simulink model "phdMain2"  (R2023b)
settings: Solver=ode4  StartTime=0.0  StopTime=t.Data(end)  FixedStep=1e-3  RelTol=1e-3
undefined symbols (not defined in the file): AEFF, Am, B_E, Bm, C_T, Cm, k, K, Kr0, Kx0, M, m3PsToLpm, PA_Pa, PaToBar, PB_Pa, PB_vec, V01, V02, V_DEAD, v_mPs, xc_dot, xc_m
(part 1 of 2)
settings Model: PauseTimes=22  Creator=snr  LastModifiedBy=snr
settings DataIOCC: OutputOption=AdditionalOutputTimes  OutputTimes=1
settings OptimizationCC: BlockReduction=off  ConditionallyExecuteInputs=off
settings DebuggingCC: UnderSpecifiedDimensionMsg=warning

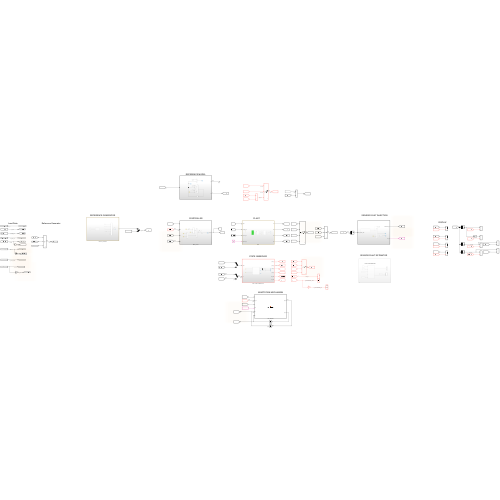
[thumbnail: Simulink's stored preview of the top-level diagram]
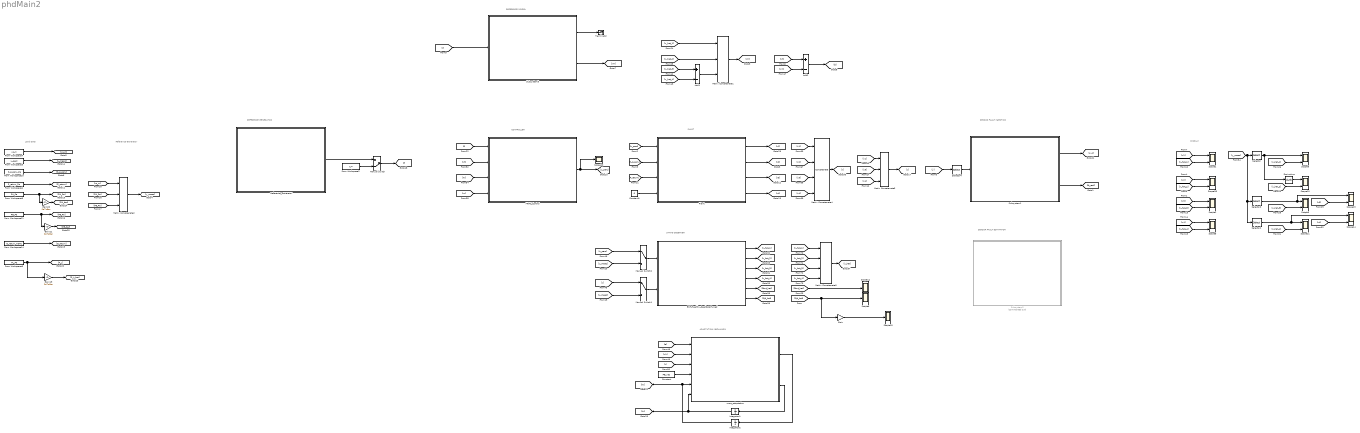
== system phdMain2 ==
  note: Load Data
  note: PLANT
  note: DISPLAY
  note: Reference Generator
  note: SENSOR FAULT INJECTION
  note: STATE OBSERVER
  note: SENSOR FAULT ESTIMATOR
  note: REFERENCE GENERATOR
  note: REFERENCE MODEL
  note: ADAPTATION MECHANISM
  note: CONTROLLER
  Add1 : Sum  Inputs=+-
  Add2 : Sum  Inputs=+-
  Constant : Constant  Value=PB_vec
  Constant1 : Constant  Value=0
  Derivative : Derivative
  EKF_Healthy_RealDataTuned : Subsystem
  From Workspace1 : FromWorkspace  VariableName=P_return_Pa
  From Workspace10 : FromWorkspace  VariableName=P_supply_Pa
  From Workspace11 : FromWorkspace  VariableName=PB_Pa
  From Workspace14 : FromWorkspace  VariableName=Q_return_m3Ps
  From Workspace2 : FromWorkspace  VariableName=r_m
  From Workspace3 : FromWorkspace  VariableName=u_perc
  From Workspace4 : FromWorkspace  VariableName=xc_m
  From Workspace5 : FromWorkspace  VariableName=PL_Pa
  From Workspace9 : FromWorkspace  VariableName=PA_Pa
  Gain : Gain  Gain=60e3
  Gain19 : Gain  Gain=PaToBar
  Gain20 : Gain  Gain=PaToBar
  Gain21 : Gain  Gain=PaToBar
  Integrator1 : Integrator  InitialCondition=Kr0
  Integrator2 : Integrator  InitialCondition=Kx0
  MRAC_Control : Subsystem
  Manual Switch : ManualSwitch  CurrentSetting=0
  Manual Switch1 : ManualSwitch
  Manual Switch2 : ManualSwitch
  Matrix Concatenate1 : Concatenate  NumInputs=3  Mode=Multidimensional array
  Matrix Concatenate2 : Concatenate  NumInputs=3  Mode=Multidimensional array
  Matrix Concatenate3 : Concatenate  NumInputs=3  Mode=Multidimensional array
  Matrix Concatenate4 : Concatenate  NumInputs=4  Mode=Multidimensional array
  Matrix Concatenate5 : Concatenate  NumInputs=4  Mode=Multidimensional array
  Plant : Subsystem
  Reference_Generator : Subsystem
  Scope{1..2,5,8..11,13..14,36} (10 alike) : Scope  NumInputPorts=2
  Scope{6,12,15,20} (4 alike) : Scope
  Selector : Selector  InputPortWidth=3  IndexOptions=Index vector (dialog)  Indices=1  OutputSizes=1
  Selector1 : Selector  InputPortWidth=3  IndexOptions=Index vector (dialog)  Indices=3  OutputSizes=1
  Selector2 : Selector  InputPortWidth=3  IndexOptions=Index vector (dialog)  Indices=2  OutputSizes=1
  Selector4 : Selector  InputPortWidth=3  IndexOptions=Index vector (dialog)  Indices=1  OutputSizes=1
  Subsystem1 : Subsystem
  Subsystem2 : Subsystem  Commented=on
  Subsystem3 : Subsystem
  Terminator : Terminator
  mrac_adaptation : MATLAB Function  TreatAsAtomicUnit=on
  wires:
  From Workspace3/1 -> [u_meas]  "u_real"
  From Workspace10/1 -> [P_supply]  "P_supply_Pa"
  From Workspace1/1 -> [P_return]  "P_return_Pa"
  From Workspace9/1 -> Gain20/1, [PA_Pa]  "PA_Pa"
  From Workspace11/1 -> Gain21/1, [PB_Pa]  "PB_Pa"
  From Workspace14/1 -> [Q_return]  "Q_return_m3Ps"
  From Workspace5/1 -> [P_L], Gain19/1  "P_L_Pa"
  Gain19/1 -> [P_L_bar]  "P_L_bar"
  Gain20/1 -> [PA_bar]  "PA_bar"
  Gain21/1 -> [PB_bar]  "PB_bar"
  [P_supply] -> Plant/2(P_supply_Pa)
  [P_return] -> Plant/3(P_return_Pa)
  Plant/1(x1) -> [x1]
  Plant/2(x2) -> [x2]
  Plant/3(x3) -> [x3]
  Plant/4(x4) -> [x4]
  [x1] -> Matrix Concatenate3/1
  [x3] -> Matrix Concatenate3/2
  [x4] -> Matrix Concatenate3/3
  Matrix Concatenate3/1 -> [y]
  EKF_Healthy_RealDataTuned/1(x_hat_1) -> [x_hat_1]  "x_hat_1"
  EKF_Healthy_RealDataTuned/2(x_hat_2) -> [x_hat_2]  "x_hat_2"
  EKF_Healthy_RealDataTuned/3(x_hat_3) -> [x_hat_3]
  EKF_Healthy_RealDataTuned/4(x_hat_4) -> [x_hat_4]
  [x1] -> Matrix Concatenate4/1
  [x2] -> Matrix Concatenate4/2
  [x3] -> Matrix Concatenate4/3
  [x4] -> Matrix Concatenate4/4
  Matrix Concatenate4/1 -> [x]
  [x_hat_1] -> Matrix Concatenate5/1
  [x_hat_2] -> Matrix Concatenate5/2
  [x_hat_3] -> Matrix Concatenate5/3
  [x_hat_4] -> Matrix Concatenate5/4
  Matrix Concatenate5/1 -> [x_hat]
  EKF_Healthy_RealDataTuned/5(Fext_hat) -> [Fext_hat]
  EKF_Healthy_RealDataTuned/6(Qd_est) -> [Qd_hat]
  [x2] -> Scope36/1
  [x_hat_2] -> Scope36/2
  [y] -> Selector4/1
  Selector4/1 -> Subsystem1/1(Real_Cylinder_Pos)
  Subsystem1/1(Measured_Pos) -> [y_1]
  Subsystem1/2(fs_real) -> [fs_real]
  [r] -> Subsystem3/1(r)  "r"
  Manual Switch/1 -> [r]  "r_m"
  Reference_Generator/1(r) -> Manual Switch/1  "r"
  From Workspace2/1 -> Manual Switch/2
  [x1] -> Scope1/1
  [x_hat_1] -> Scope1/2
  [x_hat_3] -> Scope2/2
  [x3] -> Scope2/1
  [x4] -> Scope5/1
  [x_hat_4] -> Scope5/2
  [Qd_hat] -> Gain/1, Scope6/1  "Q_unmodeledLeak_m3Ps"
  [PB_Pa] -> Matrix Concatenate2/3
  [PA_Pa] -> Matrix Concatenate2/2
  [xc_m] -> Matrix Concatenate2/1
  Matrix Concatenate2/1 -> [y_meas]
  Manual Switch1/1 -> EKF_Healthy_RealDataTuned/2(y_k)
  [y] -> Manual Switch1/1
  [y_meas] -> Manual Switch1/2
  Manual Switch2/1 -> EKF_Healthy_RealDataTuned/1(u_perc)
  [u_perc] -> Manual Switch2/1
  [u_meas] -> Manual Switch2/2
  [u_perc] -> Plant/1(u_perc)
  Selector1/1 -> Scope14/1, Scope11/1  "P2_real"
  [x_hat_4] -> Scope11/2
  Selector/1 -> Derivative/1, Scope8/1
  [x_hat_1] -> Scope8/2
  [x_hat_2] -> Scope10/2
  Derivative/1 -> Scope10/1
  [x_hat_3] -> Scope9/2
  Selector2/1 -> Scope13/1, Scope9/1  "P1_real"
  [y_meas] -> Selector1/1, Selector2/1, Selector/1
  From Workspace4/1 -> [xc_m]  "xc_m"
  [Fext_hat] -> Scope12/1  "Fext_N"
  [x3] -> Scope13/2
  [x4] -> Scope14/2
  Gain/1 -> Scope15/1  "Q_unmodeledLeak_lpm"
  Subsystem3/1(ym) -> Terminator/1
  Subsystem3/2(xm) -> [xm]
  [x_hat_3] -> Add1/1
  [x_hat_4] -> Add1/2
  Add1/1 -> Matrix Concatenate1/3  "PL_hat"
  [x_hat_2] -> Matrix Concatenate1/2  "x2_hat"
  [x_hat_1] -> Matrix Concatenate1/1  "x1_hat"
  Add2/1 -> [e]  "e"
  [xm] -> Add2/2
  Matrix Concatenate1/1 -> [xh]
  [e] -> mrac_adaptation/1(e)
  [xh] -> mrac_adaptation/2(x_hat)
  [r] -> mrac_adaptation/3(r)
  mrac_adaptation/2(Kr_dot) -> Integrator1/1
  Integrator1/1 -> [Kr], mrac_adaptation/6(Kr)
  mrac_adaptation/1(Kx_dot) -> Integrator2/1
  Integrator2/1 -> mrac_adaptation/5(Kx), [Kx]
  Constant/1 -> mrac_adaptation/4(PB)
  [r] -> MRAC_Control/1(r)
  [xx] -> MRAC_Control/4(xh)
  MRAC_Control/1(u_out_perc) -> Scope20/1, [u_perc]
  [xh] -> MRAC_Control/2(Kx)
  [Kr] -> MRAC_Control/3(Kr)
  Constant1/1 -> Plant/4(F_external_N)
  [xh] -> Add2/1

== system phdMain2/EKF_Healthy_RealDataTuned ==
  u_perc : Inport  OutDataTypeStr=double
  y_k : Inport  Port=2  OutDataTypeStr=double
  EKF_Discrete : MATLAB Function  TreatAsAtomicUnit=on  SystemSampleTime=1e-3
  Sel_d10 : Selector  InputPortWidth=6  IndexOptions=Index vector (dialog)  Indices=4  OutputSizes=1
  Sel_d7 : Selector  InputPortWidth=6  IndexOptions=Index vector (dialog)  Indices=1  OutputSizes=1
  Sel_d8 : Selector  InputPortWidth=6  IndexOptions=Index vector (dialog)  Indices=2  OutputSizes=1  RuntimeRangeChecks=on
  Sel_d9 : Selector  InputPortWidth=6  IndexOptions=Index vector (dialog)  Indices=3  OutputSizes=1
  Unit Delay : UnitDelay  SampleTime=1e-3  HasFrameUpgradeWarning=on
  x_hat_1 : Outport  OutDataTypeStr=double
  x_hat_2 : Outport  Port=2  OutDataTypeStr=double
  x_hat_3 : Outport  Port=3  OutDataTypeStr=double
  x_hat_4 : Outport  Port=4  OutDataTypeStr=double
  Fext_hat : Outport  Port=5  OutDataTypeStr=double
  Qd_est : Outport  Port=6  OutDataTypeStr=double
  wires:
  u_perc/1 -> EKF_Discrete/1(u_perc)  "u_perc"
  y_k/1 -> EKF_Discrete/2(y_k)
  EKF_Discrete/1(x_hat_out) -> Unit Delay/1
  Sel_d7/1 -> x_hat_1/1  "x_hat_1"
  Sel_d8/1 -> x_hat_2/1  "x_hat_2"
  Sel_d9/1 -> x_hat_3/1  "x_hat_3"
  Sel_d10/1 -> x_hat_4/1  "x_hat_4"
  EKF_Discrete/2(Fd_est) -> Fext_hat/1
  EKF_Discrete/3(Qd_est) -> Qd_est/1
  Unit Delay/1 -> Sel_d7/1, Sel_d10/1, Sel_d9/1, Sel_d8/1

== system phdMain2/MRAC_Control ==
  r : Inport  OutDataTypeStr=double
  Kx : Inport  Port=2  OutDataTypeStr=double
  Kr : Inport  Port=3  OutDataTypeStr=double
  xh : Inport  Port=4  OutDataTypeStr=double
  Add : Sum
  Product : Product  Multiplication=Matrix(*)
  Product1 : Product  Multiplication=Matrix(*)
  Saturation : Saturate  UpperLimit=100  LowerLimit=-100
  Scope : Scope
  Transpose : Math  Operator=transpose
  u_out_perc : Outport  OutDataTypeStr=double
  wires:
  xh/1 -> Product/2
  Kx/1 -> Transpose/1
  Transpose/1 -> Product/1
  r/1 -> Product1/2
  Kr/1 -> Product1/1
  Product1/1 -> Add/2
  Product/1 -> Add/1
  Add/1 -> Scope/1, Saturation/1
  Saturation/1 -> u_out_perc/1

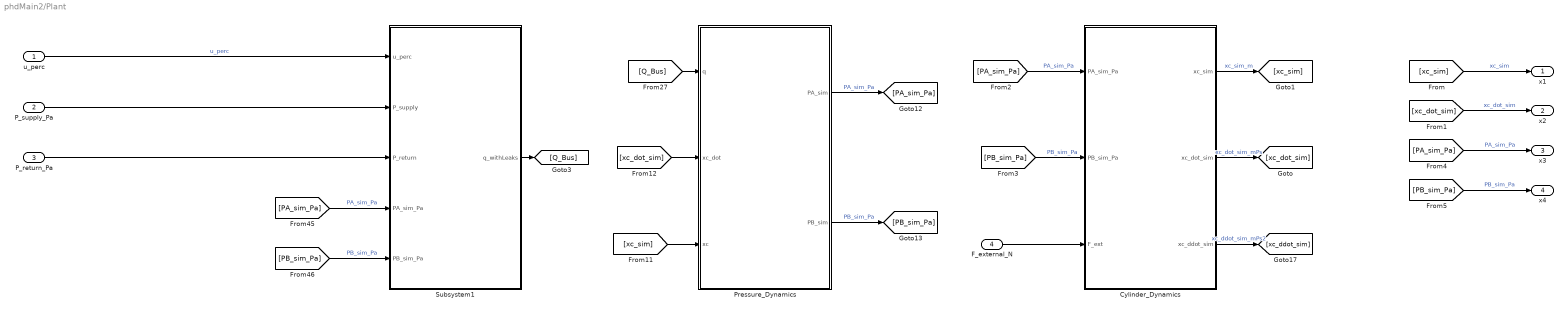
== system phdMain2/Plant ==
  u_perc : Inport  OutDataTypeStr=double
  P_supply_Pa : Inport  Port=2
  P_return_Pa : Inport  Port=3
  F_external_N : Inport  Port=4
  Cylinder_Dynamics : Subsystem
  Pressure_Dynamics : Subsystem
  Subsystem1 : Subsystem
  x1 : Outport
  x2 : Outport  Port=2
  x3 : Outport  Port=3
  x4 : Outport  Port=4
  wires:
  Cylinder_Dynamics/1(xc_sim) -> [xc_sim]  "xc_sim_m"
  [xc_sim] -> Pressure_Dynamics/3(xc)
  P_supply_Pa/1 -> Subsystem1/2(P_supply)
  [PA_sim_Pa] -> Subsystem1/4(PA_sim_Pa)  "PA_sim_Pa"
  [PB_sim_Pa] -> Subsystem1/5(PB_sim_Pa)  "PB_sim_Pa"
  [PB_sim_Pa] -> Cylinder_Dynamics/2(PB_sim_Pa)  "PB_sim_Pa"
  Pressure_Dynamics/1(PA_sim) -> [PA_sim_Pa]  "PA_sim_Pa"
  Cylinder_Dynamics/3(xc_ddot_sim) -> [xc_ddot_sim]  "xc_ddot_sim_mPs2"
  Cylinder_Dynamics/2(xc_dot_sim) -> [xc_dot_sim]  "xc_dot_sim_mPs"
  [xc_dot_sim] -> Pressure_Dynamics/2(xc_dot)
  [PA_sim_Pa] -> Cylinder_Dynamics/1(PA_sim_Pa)  "PA_sim_Pa"
  Pressure_Dynamics/2(PB_sim) -> [PB_sim_Pa]  "PB_sim_Pa"
  Subsystem1/1(q_withLeaks) -> [Q_Bus]
  [Q_Bus] -> Pressure_Dynamics/1(q)
  u_perc/1 -> Subsystem1/1(u_perc)  "u_perc"
  P_return_Pa/1 -> Subsystem1/3(P_return)
  F_external_N/1 -> Cylinder_Dynamics/3(F_ext)
  [xc_sim] -> x1/1  "xc_sim"
  [xc_dot_sim] -> x2/1  "xc_dot_sim"
  [PA_sim_Pa] -> x3/1  "PA_sim_Pa"
  [PB_sim_Pa] -> x4/1  "PB_sim_Pa"

== system phdMain2/Reference_Generator ==
  Constant : Constant  OutDataTypeStr=uint8
  Constant1 : Constant  Commented=on  Value=30  OutDataTypeStr=double
  Constant2 : Constant  Commented=on  OutDataTypeStr=double
  Constant3 : Constant  Commented=on  Value=0  OutDataTypeStr=double
  Constant4 : Constant  Value=0
  From Workspace14 : FromWorkspace  VariableName=r_m
  Gain : Gain
  Multiport Switch : MultiPortSwitch  DataPortOrder=Zero-based contiguous  DataPortForDefault=Additional data port  DiagnosticForDefault=None  zeroidx=on  OutDataTypeStr=double  SaturateOnIntegerOverflow=off  InputSameDT=off
  Pulse Generator : DiscretePulseGenerator  PulseType=Time based  Amplitude=20e-3  Period=4  PulseWidth=25
  Scope : Scope
  Sine Wave : Sin  Amplitude=30e-3  Frequency=pi*0.5  SampleTime=0
  Sine_Generator : Subsystem  Commented=on
  r : Outport  OutDataTypeStr=double
  wires:
  From Workspace14/1 -> Multiport Switch/2  "r_m"
  Constant/1 -> Multiport Switch/1
  Constant1/1 -> Sine_Generator/1(Amp_mm)
  Constant2/1 -> Sine_Generator/2(f_Hz)
  Constant3/1 -> Sine_Generator/3(phi_deg)
  Pulse Generator/1 -> Gain/1
  Multiport Switch/1 -> Scope/1, r/1
  Constant4/1 -> Multiport Switch/5
  Sine Wave/1 -> Multiport Switch/3
  Gain/1 -> Multiport Switch/4

== system phdMain2/Subsystem1 ==
  Real_Cylinder_Pos : Inport  OutDataTypeStr=double
  Add4 : Sum
  Fault_Injection : Subsystem  Commented=on
  Measured_Pos : Outport  OutDataTypeStr=double
  fs_real : Outport  Port=2  OutDataTypeStr=double
  wires:
  Fault_Injection/1(fs) -> [fs_real], Add4/1
  Real_Cylinder_Pos/1 -> Add4/2
  Add4/1 -> Measured_Pos/1  "y_1"
  [fs_real] -> fs_real/1

== system phdMain2/Subsystem2 ==
  note: FAULT ESTIMATOR
  From14 : From  Commented=on  GotoTag=u_perc
  From15 : From  Commented=on  GotoTag=PA_sim_Pa
  From20 : From  Commented=on  GotoTag=PB_sim_Pa
  From29 : From  Commented=on  GotoTag=fs_real
  From33 : From  Commented=on  GotoTag=xc_dot_sim
  Scope12 : Scope  Commented=on  NumInputPorts=3
  Scope17 : Scope  Commented=on  NumInputPorts=3
  Subsystem3 : Subsystem  Commented=on
  wires:
  Subsystem3/2(Out1) -> Scope17/1
  From20/1 -> Subsystem3/3(PB_Pa)  "PB_sim_Pa"
  From29/1 -> Subsystem3/5(fs_real)
  From14/1 -> Subsystem3/1(u_real)  "u_perc"
  From33/1 -> Scope17/2
  From15/1 -> Subsystem3/2(PA_Pa)
  Subsystem3/1(x_bar) -> Scope12/2  "x_bar"

== system phdMain2/Subsystem3 ==
  r : Inport  OutDataTypeStr=double
  Add : Sum
  Constant : Constant  Value=Am
  Constant1 : Constant  Value=Bm
  Constant2 : Constant  Value=Cm
  Integrator1 : Integrator  InitialCondition=[0;0;0]
  Product : Product  Multiplication=Matrix(*)
  Product1 : Product  Multiplication=Matrix(*)
  Product2 : Product  Multiplication=Matrix(*)
  ym : Outport  OutDataTypeStr=double  PortDimensions=[3,1]
  xm : Outport  Port=2  OutDataTypeStr=double
  wires:
  Constant/1 -> Product/1
  Constant1/1 -> Product1/1
  r/1 -> Product1/2  "r"
  Product1/1 -> Add/2
  Product/1 -> Add/1
  Add/1 -> Integrator1/1  "dxm"
  Integrator1/1 -> Product/2, Product2/2, xm/1  "xm"
  Product2/1 -> ym/1
  Constant2/1 -> Product2/1

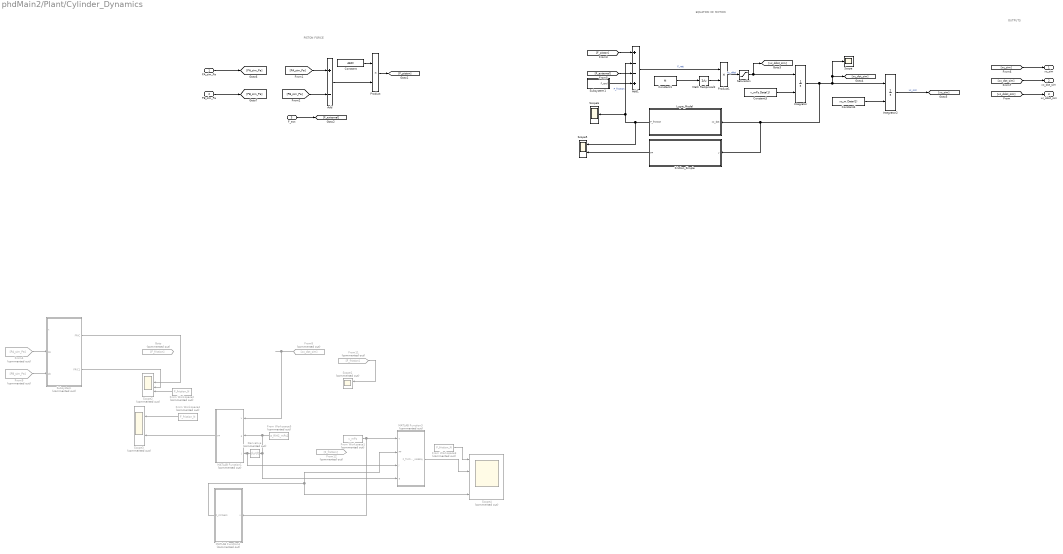
== system phdMain2/Plant/Cylinder_Dynamics ==
  note: PISTON FORCE
  note: EQUATION OF MOTION
  note: OUTPUTS
  PA_sim_Pa : Inport  OutDataTypeStr=double
  PB_sim_Pa : Inport  Port=2  OutDataTypeStr=double
  F_ext : Inport  Port=3  OutDataTypeStr=double
  Add : Sum  Inputs=+-
  Add1 : Sum  Inputs=+--+
  Constant : Constant  Value=AEFF  OutDataTypeStr=double
  Constant1 : Constant  Value=M  OutDataTypeStr=double
  Constant3 : Constant  Value=v_mPs.Data(1)
  Constant4 : Constant  Value=xc_m.Data(1)
  Derivative : Derivative  Commented=on
  Friction_Simple : MATLAB Function  TreatAsAtomicUnit=on
  From Workspace1 : FromWorkspace  Commented=on  VariableName=v_mPs
  From Workspace2 : FromWorkspace  Commented=on  VariableName=F_friction_N
  From Workspace3 : FromWorkspace  Commented=on  VariableName=F_friction_N
  From Workspace4 : FromWorkspace  Commented=on  VariableName=F_friction_N
  From Workspace5 : FromWorkspace  Commented=on  VariableName=a_RMC_mPs2
  From11 : From  Commented=on  GotoTag=F_friction
  From12 : From  Commented=on  GotoTag=F_friction
  From4 : From  Commented=on  GotoTag=PA_sim_Pa
  From8 : From  Commented=on  GotoTag=xc_dot_sim
  From9 : From  Commented=on  GotoTag=PB_sim_Pa
  Goto : Goto  Commented=on  GotoTag=F_friction
  Integrator : Integrator  InitialConditionSource=external  InitialCondition=xc_dot(1)  UpperSaturationLimit=4  LowerSaturationLimit=-4
  Integrator2 : Integrator  InitialConditionSource=external  InitialCondition=xc_dot(1)  LimitOutput=on  UpperSaturationLimit=0.09580  LowerSaturationLimit=-0.09580
  Lugre_Model : Subsystem
  MATLAB Function1 : MATLAB Function  Commented=on  TreatAsAtomicUnit=on
  MATLAB Function3 : MATLAB Function  Commented=on  TreatAsAtomicUnit=on
  MATLAB Function4 : MATLAB Function  Commented=on  TreatAsAtomicUnit=on
  Math Reciprocal2 : Math  Operator=reciprocal  SignedPower=on
  Product : Product
  Product1 : Product
  Saturation : Saturate  UpperLimit=100  LowerLimit=-100
  Scope : Scope
  Scope1 : Scope  Commented=on  NumInputPorts=2
  Scope2 : Scope  Commented=on  NumInputPorts=6
  Scope3 : Scope  Commented=on  NumInputPorts=2
  Scope4 : Scope  Commented=on  NumInputPorts=4
  Scope5 : Scope  NumInputPorts=2
  Scope6 : Scope
  Subsystem : Subsystem  Commented=on
  Subsystem1 : Subsystem
  xc_sim : Outport  OutDataTypeStr=double
  xc_dot_sim : Outport  Port=2  OutDataTypeStr=double
  xc_ddot_sim : Outport  Port=3  OutDataTypeStr=double
  wires:
  [PB_sim_Pa] -> Add/2
  [PA_sim_Pa] -> Add/1
  Add/1 -> Product/2
  Constant/1 -> Product/1
  Math Reciprocal2/1 -> Product1/2
  Product1/1 -> Saturation/1  "xc_ddot"
  Product/1 -> [F_piston]
  F_ext/1 -> [F_external]
  Add1/1 -> Product1/1  "F_net"
  Constant3/1 -> Integrator/2
  Integrator/1 -> Integrator2/1, Scope/1, [xc_dot_sim], Friction_Simple/1(v), Lugre_Model/1(xc_dot)
  Constant4/1 -> Integrator2/2
  Integrator2/1 -> [xc_sim]  "xc_sim"
  [xc_sim] -> xc_sim/1
  [xc_dot_sim] -> xc_dot_sim/1
  From8/1 -> MATLAB Function1/1(v)
  [xc_ddot_sim] -> xc_ddot_sim/1
  Saturation/1 -> [xc_ddot_sim], Integrator/1
  [F_external] -> Add1/3
  [F_piston] -> Add1/1
  ? -> Scope2/1, Goto/1  "F_friction"
  From Workspace2/1 -> Scope2/5
  Subsystem1/1(F_end) -> Add1/4
  PA_sim_Pa/1 -> [PA_sim_Pa]
  PB_sim_Pa/1 -> [PB_sim_Pa]
  From4/1 -> Subsystem/2(pa)
  From9/1 -> Subsystem/3(pb)
  Constant1/1 -> Math Reciprocal2/1
  Subsystem/2(FRIC1) -> Scope2/4
  Subsystem/1(FRIC) -> Scope2/3
  Derivative/1 -> MATLAB Function3/3(j), MATLAB Function1/3(j)
  From Workspace4/1 -> Scope3/1
  MATLAB Function1/1(FF) -> Scope3/2
  From Workspace5/1 -> MATLAB Function3/4(a), Derivative/1, MATLAB Function1/2(a)
  From11/1 -> Scope1/1
  From Workspace1/1 -> MATLAB Function4/1(v), MATLAB Function3/1(v)
  MATLAB Function3/1(F_friction_nodelay) -> Scope4/2
  From Workspace3/1 -> Scope4/1
  MATLAB Function4/1(F_stribeck) -> MATLAB Function3/2(FF), Scope4/4
  Lugre_Model/1(F_friction) -> Add1/2, Scope6/1, Scope5/1  "F_friction"
  Friction_Simple/1(FF) -> Scope5/2

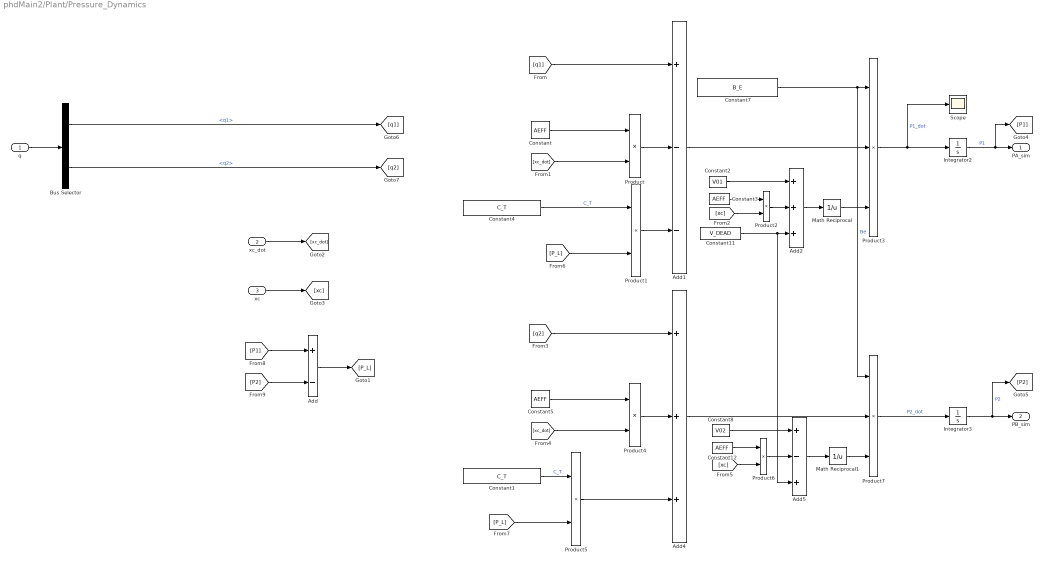
== system phdMain2/Plant/Pressure_Dynamics ==
  q : Inport  OutDataTypeStr=double
  xc_dot : Inport  Port=2  OutDataTypeStr=double
  xc : Inport  Port=3  OutDataTypeStr=double
  Add : Sum  Inputs=+-
  Add1 : Sum  Inputs=+--
  Add2 : Sum  Inputs=+++
  Add4 : Sum  Inputs=+++
  Add5 : Sum  Inputs=+-+
  Bus Selector : BusSelector  OutputSignals=q1,q2
  Constant{,3,5,12} (4 alike) : Constant  Value=AEFF  OutDataTypeStr=double
  Constant1 : Constant  Value=C_T  OutDataTypeStr=double
  Constant11 : Constant  Value=V_DEAD  OutDataTypeStr=double
  Constant2 : Constant  Value=V01  OutDataTypeStr=double
  Constant4 : Constant  Value=C_T  OutDataTypeStr=double
  Constant7 : Constant  Value=B_E  OutDataTypeStr=double
  Constant8 : Constant  Value=V02  OutDataTypeStr=double
  Integrator2 : Integrator  InitialCondition=PA_Pa.Data(1)  LimitOutput=on  UpperSaturationLimit=200e5  LowerSaturationLimit=4e5
  Integrator3 : Integrator  InitialCondition=PB_Pa.Data(1)  LimitOutput=on  UpperSaturationLimit=200e5  LowerSaturationLimit=4e5
  Math Reciprocal : Math  Operator=reciprocal  SignedPower=on
  Math Reciprocal1 : Math  Operator=reciprocal  SignedPower=on
  Product{,1..2,4..6} (6 alike) : Product
  Product3 : Product  Inputs=3
  Product7 : Product  Inputs=3
  Scope : Scope
  PA_sim : Outport  OutDataTypeStr=double
  PB_sim : Outport  Port=2  OutDataTypeStr=double
  wires:
  q/1 -> Bus Selector/1
  xc_dot/1 -> [xc_dot]
  [xc_dot] -> Product/2
  Constant/1 -> Product/1
  Integrator2/1 -> [P1], PA_sim/1  "P1"
  [P_L] -> Product1/2
  Product/1 -> Add1/2
  [q1] -> Add1/1
  xc/1 -> [xc]
  Constant2/1 -> Add2/1
  Product2/1 -> Add2/2
  [xc] -> Product2/2
  Constant3/1 -> Product2/1
  Add2/1 -> Math Reciprocal/1
  Product3/1 -> Integrator2/1, Scope/1  "P1_dot"
  Math Reciprocal/1 -> Product3/3
  Add1/1 -> Product3/2
  Constant7/1 -> Product7/1, Product3/1  "Be"
  Constant4/1 -> Product1/1  "C_T"
  [xc_dot] -> Product4/2
  Product4/1 -> Add4/2
  Add4/1 -> Product7/2
  Integrator3/1 -> [P2], PB_sim/1  "P2"
  [P_L] -> Product5/2
  Constant5/1 -> Product4/1
  Add5/1 -> Math Reciprocal1/1
  [q2] -> Add4/1
  Math Reciprocal1/1 -> Product7/3
  Product7/1 -> Integrator3/1  "P2_dot"
  [xc] -> Product6/2
  Constant8/1 -> Add5/1
  Constant12/1 -> Product6/1
  Product6/1 -> Add5/2
  Bus Selector/2 -> [q2]  "<q2>"
  Bus Selector/1 -> [q1]  "<q1>"
  [P2] -> Add/2
  [P1] -> Add/1
  Add/1 -> [P_L]
  Constant1/1 -> Product5/1  "C_T"
  Product5/1 -> Add4/3
  Product1/1 -> Add1/3
  Constant11/1 -> Add5/3, Add2/3

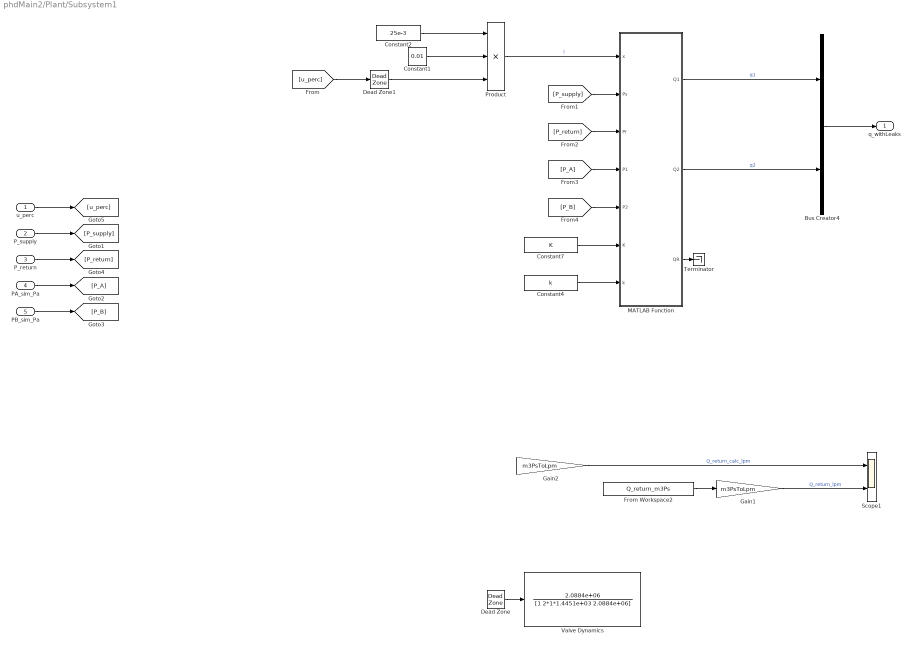
== system phdMain2/Plant/Subsystem1 ==
  u_perc : Inport  OutDataTypeStr=double
  P_supply : Inport  Port=2  OutDataTypeStr=double
  P_return : Inport  Port=3  OutDataTypeStr=double
  PA_sim_Pa : Inport  Port=4  OutDataTypeStr=double
  PB_sim_Pa : Inport  Port=5  OutDataTypeStr=double
  Bus Creator4 : BusCreator  Inputs=2
  Constant1 : Constant  Value=0.01
  Constant2 : Constant  Value=25e-3
  Constant4 : Constant  Value=k
  Constant7 : Constant  Value=K
  Dead Zone : DeadZone  LowerValue=-0.02  UpperValue=0.02
  Dead Zone1 : DeadZone  LowerValue=-0.02  UpperValue=0.02
  From Workspace2 : FromWorkspace  VariableName=Q_return_m3Ps
  Gain1 : Gain  Gain=m3PsToLpm
  Gain2 : Gain  Gain=m3PsToLpm
  MATLAB Function : MATLAB Function  TreatAsAtomicUnit=on
  Product : Product  Inputs=3
  Scope1 : Scope  NumInputPorts=2
  Terminator : Terminator
  Valve Dynamics : TransferFcn  Numerator=[2.0884e+06]  Denominator=[1 2*1*1.4451e+03 2.0884e+06]
  q_withLeaks : Outport  OutDataTypeStr=double
  wires:
  PA_sim_Pa/1 -> [P_A]
  P_supply/1 -> [P_supply]
  P_return/1 -> [P_return]
  PB_sim_Pa/1 -> [P_B]
  u_perc/1 -> [u_perc]
  [P_supply] -> MATLAB Function/2(Ps)
  [P_return] -> MATLAB Function/3(Pr)
  [P_A] -> MATLAB Function/4(P1)
  [P_B] -> MATLAB Function/5(P2)
  Bus Creator4/1 -> q_withLeaks/1
  MATLAB Function/1(Q1) -> Bus Creator4/1  "q1"
  MATLAB Function/2(Q2) -> Bus Creator4/2  "q2"
  Constant2/1 -> Product/1
  Product/1 -> MATLAB Function/1(x)  "i"
  Constant1/1 -> Product/2
  Constant4/1 -> MATLAB Function/7(k)
  Constant7/1 -> MATLAB Function/6(K)
  [u_perc] -> Dead Zone1/1
  From Workspace2/1 -> Gain1/1
  Gain2/1 -> Scope1/1  "Q_return_calc_lpm"
  Gain1/1 -> Scope1/2  "Q_return_lpm"
  MATLAB Function/3(QR) -> Terminator/1
  Dead Zone/1 -> Valve Dynamics/1
  Dead Zone1/1 -> Product/3

== system phdMain2/Reference_Generator/Sine_Generator ==
  Amp_mm : Inport  OutDataTypeStr=double
  f_Hz : Inport  Port=2
  phi_deg : Inport  Port=3  OutDataTypeStr=double
  Add : Sum
  Clock : Clock
  Constant : Constant  Value=2
  Constant1 : Constant  Value=3.14159265359
  Constant2 : Constant  Value=3.14159265359
  Constant3 : Constant  Value=180
  Constant4 : Constant  Value=1e-3
  Math Reciprocal : Math  Operator=reciprocal  SignedPower=on
  Product : Product  Inputs=4
  Product{1..4} (4 alike) : Product
  Sin : Trigonometry
  r : Outport
  wires:
  Constant1/1 -> Product/2
  Constant/1 -> Product/1
  f_Hz/1 -> Product/3
  phi_deg/1 -> Product1/1
  Constant2/1 -> Product2/1
  Constant3/1 -> Math Reciprocal/1
  Math Reciprocal/1 -> Product2/2
  Product2/1 -> Product1/2
  Clock/1 -> Product/4
  Product/1 -> Sin/1
  Sin/1 -> Product3/2
  Product1/1 -> Add/2
  Product3/1 -> Add/1
  Add/1 -> r/1
  Amp_mm/1 -> Product4/2
  Product4/1 -> Product3/1
  Constant4/1 -> Product4/1

== system phdMain2/Subsystem1/Fault_Injection ==
  Constant : Constant  Value=0
  fs : Outport  OutDataTypeStr=double
  wires:
  Constant/1 -> fs/1

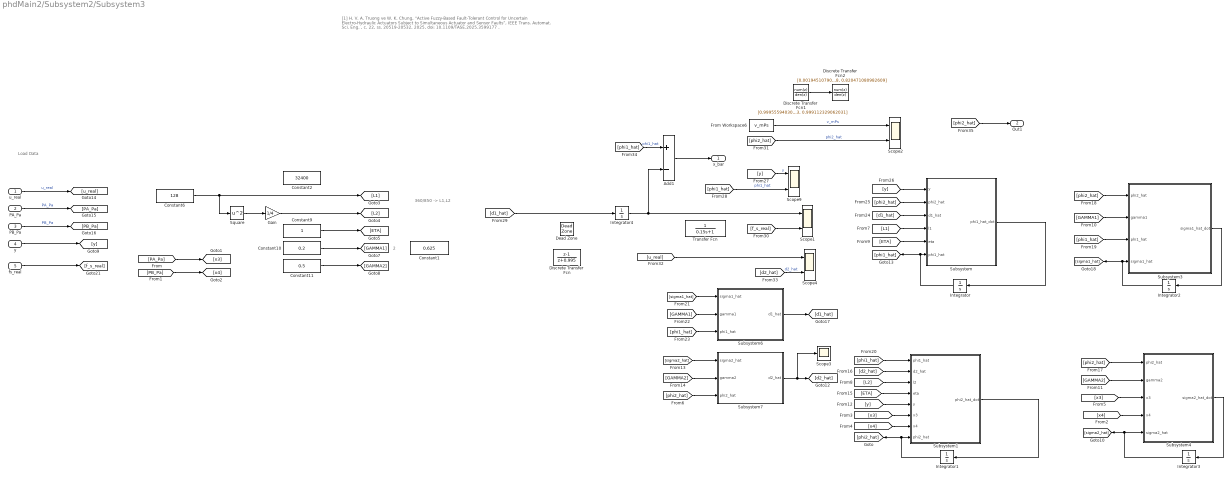
== system phdMain2/Subsystem2/Subsystem3 ==
  note: [1]
      | H. V. A. Truong ve W. K. Chung, “Active Fuzzy-Based Fault-Tolerant Control for Uncertain Electro-Hydraulic Actuators Subject to Simultaneous Actuator and Sensor Faults”, IEEE Trans. Automat. Sci. Eng. , c. 22, ss. 20519-20532, 2025, doi: 10.1109/TASE.2025.3599177 .
  note: 2
  note: 360/850 -> L1,L2
  note: Load Data
  u_real : Inport
  PA_Pa : Inport  Port=2
  PB_Pa : Inport  Port=3
  y : Inport  Port=4
  fs_real : Inport  Port=5
  Add1 : Sum  Inputs=+-
  Constant1 : Constant  Value=0.625
  Constant10 : Constant  Value=0.2
  Constant11 : Constant  Value=0.5
  Constant2 : Constant  Value=32400
  Constant6 : Constant  Value=128
  Constant9 : Constant
  Dead Zone : DeadZone  LowerValue=-0.01  UpperValue=0.01
  Discrete Transfer Fcn : DiscreteTransferFcn  Numerator=[1 -1]  Denominator=[1 0.995]
  Discrete Transfer Fcn1 : DiscreteTransferFcn  Numerator=[0.999555940307616, -1.999111880615232, 0.999555940307616]  Denominator=[1.000000000000000, -1.999111432168433, 0.999112329062031]
  Discrete Transfer Fcn2 : DiscreteTransferFcn  Numerator=[0.001945107908955, 0.003890215817911, 0.001945107908955]  Denominator=[1.000000000000000, -1.812690649346788, 0.820471080982609]
  From Workspace6 : FromWorkspace  VariableName=v_mPs
  Gain : Gain  Gain=1/4
  Integrator{,1..4} (5 alike) : Integrator
  Scope{1..2,4,9} (4 alike) : Scope  NumInputPorts=2
  Scope3 : Scope
  Square : Math  Operator=square
  Subsystem : Subsystem
  Subsystem1 : Subsystem
  Subsystem3 : Subsystem
  Subsystem4 : Subsystem
  Subsystem6 : Subsystem
  Subsystem7 : Subsystem
  Transfer Fcn : TransferFcn  Denominator=[0.15 1]
  x_bar : Outport
  Out1 : Outport  Port=2
  wires:
  [u_real] -> Scope4/1
  Subsystem4/1(sigma2_hat_dot) -> Integrator3/1
  Constant6/1 -> Square/1, [L1]
  [y] -> Subsystem/1(y)
  Constant9/1 -> [ETA]
  [GAMMA2] -> Subsystem7/2(gamma2)
  [GAMMA1] -> Subsystem3/2(gamma1)
  Subsystem/1(phi1_hat_dot) -> Integrator/1
  Gain/1 -> [L2]
  [GAMMA1] -> Subsystem6/2(gamma1)
  [y] -> Subsystem1/5(y)
  Constant10/1 -> [GAMMA1]
  y/1 -> [y]
  [GAMMA2] -> Subsystem4/2(gamma2)
  Subsystem7/1(d2_hat) -> Scope3/1, [d2_hat]
  [L2] -> Subsystem1/3(l2)
  Subsystem6/1(d1_hat) -> [d1_hat]
  [phi1_hat] -> Subsystem3/3(phi1_hat)
  [ETA] -> Subsystem/5(eta)
  [phi1_hat] -> Scope9/2  "phi1_hat"
  Integrator/1 -> [phi1_hat], Subsystem/6(phi1_hat)
  [d2_hat] -> Subsystem1/2(d2_hat)
  Constant11/1 -> [GAMMA2]
  [d2_hat] -> Scope4/2  "d2_hat"
  [phi2_hat] -> Subsystem7/3(phi2_hat)
  [y] -> Scope9/1  "y"
  [phi2_hat] -> Subsystem4/1(phi2_hat)
  [sigma1_hat] -> Subsystem6/1(sigma1_hat)
  [L1] -> Subsystem/4(l1)
  Integrator2/1 -> [sigma1_hat], Subsystem3/4(sigma1_hat)
  [PA_Pa] -> [x3]
  [x3] -> Subsystem1/6(x3)
  PB_Pa/1 -> [PB_Pa]  "PB_Pa"
  u_real/1 -> [u_real]  "u_real"
  Subsystem3/1(sigma1_hat_dot) -> Integrator2/1
  [ETA] -> Subsystem1/4(eta)
  [phi1_hat] -> Subsystem6/3(phi1_hat)
  Integrator3/1 -> Subsystem4/5(sigma2_hat), [sigma2_hat]
  [sigma2_hat] -> Subsystem7/1(sigma2_hat)
  [x3] -> Subsystem4/3(x3)
  [x4] -> Subsystem4/4(x4)
  [d1_hat] -> Subsystem/3(d1_hat)
  From Workspace6/1 -> Scope2/1  "v_mPs"
  [phi1_hat] -> Subsystem1/1(phi1_hat)
  [phi2_hat] -> Subsystem/2(phi2_hat)
  [phi2_hat] -> Subsystem3/1(phi2_hat)
  [x4] -> Subsystem1/7(x4)
  PA_Pa/1 -> [PA_Pa]  "PA_Pa"
  [PB_Pa] -> [x4]
  [phi1_hat] -> Add1/1  "phi1_hat"
  Add1/1 -> x_bar/1
  fs_real/1 -> [f_s_real]
  [phi2_hat] -> Out1/1
  Subsystem1/1(phi2_hat_dot) -> Integrator1/1
  Integrator1/1 -> Subsystem1/8(phi2_hat), [phi2_hat]
  Square/1 -> Gain/1
  [d1_hat] -> Integrator4/1
  Integrator4/1 -> Scope1/1, Add1/2
  [f_s_real] -> Scope1/2
  Discrete Transfer Fcn1/1 -> Discrete Transfer Fcn2/1
  [phi2_hat] -> Scope2/2  "phi2_hat"

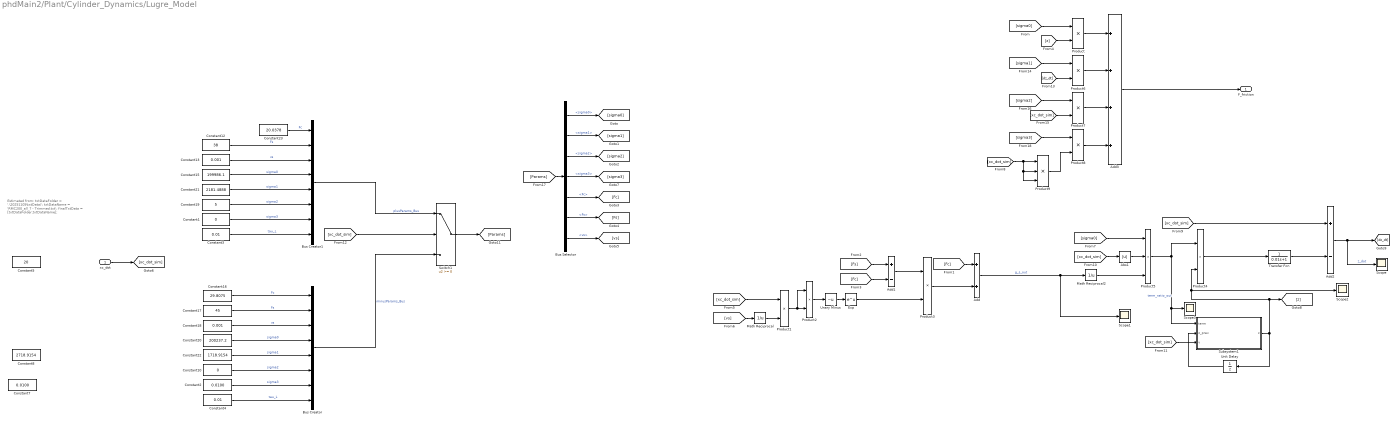
== system phdMain2/Plant/Cylinder_Dynamics/Lugre_Model ==
  note: Estimated from:
      |
      | txtDataFolder = '.\20251105\txtData\';
      | txtDataName = 'RMC200_all_7 - Trimmed.txt';
      | finalTxtData = [txtDataFolder,txtDataName];
  xc_dot : Inport  OutDataTypeStr=double
  Abs1 : Abs  SaturateOnIntegerOverflow=off
  Add : Sum
  Add1 : Sum  Inputs=+-
  Add2 : Sum  Inputs=+-
  Add3 : Sum  Inputs=++++
  Bus Selector : BusSelector  OutputSignals=sigma0,sigma1,sigma2,sigma3,Fc,Fs,vs
  Bus Creator : BusCreator  Inputs=8
  Bus Creator1 : BusCreator  Inputs=8
  Constant1 : Constant  Value=0  OutDataTypeStr=double
  Constant10 : Constant  Value=0  OutDataTypeStr=double
  Constant12 : Constant  Value=38  OutDataTypeStr=double
  Constant13 : Constant  Value=0.001  OutDataTypeStr=double
  Constant15 : Constant  Value=199986.1  OutDataTypeStr=double
  Constant16 : Constant  Value=29.8075  OutDataTypeStr=double
  Constant17 : Constant  Value=45  OutDataTypeStr=double
  Constant18 : Constant  Value=0.001  OutDataTypeStr=double
  Constant19 : Constant  Value=5  OutDataTypeStr=double
  Constant2 : Constant  Value=0.0100  OutDataTypeStr=double
  Constant20 : Constant  Value=200237.2  OutDataTypeStr=double
  Constant21 : Constant  Value=2181.4888  OutDataTypeStr=double
  Constant22 : Constant  Value=1718.9154  OutDataTypeStr=double
  Constant23 : Constant  Value=20.0378  OutDataTypeStr=double
  Constant3 : Constant  Value=0.01  OutDataTypeStr=double
  Constant4 : Constant  Value=0.01  OutDataTypeStr=double
  Constant5 : Constant  Value=20  OutDataTypeStr=double
  Constant7 : Constant  Value=0.0100  OutDataTypeStr=double
  Constant8 : Constant  Value=2718.9154  OutDataTypeStr=double
  Exp : Math  SignedPower=on
  Math Reciprocal : Math  Operator=reciprocal  SignedPower=on
  Math Reciprocal2 : Math  Operator=reciprocal  SignedPower=on
  Product{,1..4,6..8} (8 alike) : Product
  Product5 : Product  Inputs=3
  Product9 : Product  Inputs=3
  Scope{,1..3} (4 alike) : Scope
  Subsystem1 : Subsystem
  Switch1 : Switch  SaturateOnIntegerOverflow=off  InputSameDT=off
  Transfer Fcn : TransferFcn  Denominator=[0.01 1]
  Unary Minus : UnaryMinus
  Unit Delay : UnitDelay  SampleTime=-1  HasFrameUpgradeWarning=on
  F_friction : Outport
  wires:
  Constant18/1 -> Bus Creator/3  "vs"
  Constant13/1 -> Bus Creator1/3  "vs"
  Constant12/1 -> Bus Creator1/2  "Fs"
  Constant17/1 -> Bus Creator/2  "Fs"
  Constant22/1 -> Bus Creator/5  "sigma1"
  Constant20/1 -> Bus Creator/4  "sigma0"
  Constant10/1 -> Bus Creator/6  "sigma2"
  Constant16/1 -> Bus Creator/1  "Fc"
  Constant21/1 -> Bus Creator1/5  "sigma1"
  Constant15/1 -> Bus Creator1/4  "sigma0"
  Constant19/1 -> Bus Creator1/6  "sigma2"
  Product7/1 -> Add3/3
  Product6/1 -> Add3/2
  [sigma2] -> Product7/1
  [xc_dot_sim] -> Product7/2
  [dz_dt] -> Product6/2
  [sigma1] -> Product6/1
  Product/1 -> Add3/1
  [z] -> Product/2
  [sigma0] -> Product5/1
  Abs1/1 -> Product5/2
  Add/1 -> Math Reciprocal2/1, Scope1/1  "g_s_out"
  [xc_dot_sim] -> Abs1/1
  Add1/1 -> Product3/1
  Unary Minus/1 -> Exp/1
  Product2/1 -> Unary Minus/1
  Product1/1 -> Product2/2, Product2/1
  [xc_dot_sim] -> Product1/1
  Math Reciprocal/1 -> Product1/2
  [vs] -> Math Reciprocal/1
  [Fc] -> Add1/2
  [Fs] -> Add1/1
  [Fc] -> Add/1
  [sigma0] -> Product/1
  Product3/1 -> Add/2
  Bus Creator1/1 -> Switch1/1  "plusParams_Bus"
  Bus Creator/1 -> Switch1/3  "minusParams_Bus"
  [Params] -> Bus Selector/1
  Bus Selector/1 -> [sigma0]  "<sigma0>"
  Bus Selector/2 -> [sigma1]  "<sigma1>"
  Bus Selector/3 -> [sigma2]  "<sigma2>"
  Bus Selector/5 -> [Fc]  "<Fc>"
  Bus Selector/6 -> [Fs]  "<Fs>"
  Bus Selector/7 -> [vs]  "<vs>"
  Math Reciprocal2/1 -> Product5/3
  Exp/1 -> Product3/2
  Add2/1 -> Scope/1, [dz_dt]  "z_dot"
  [xc_dot_sim] -> Switch1/2
  [xc_dot_sim] -> Add2/1
  [xc_dot_sim] -> Subsystem1/3(v)
  Unit Delay/1 -> Subsystem1/2(z_prev)
  Product5/1 -> Scope3/1, Subsystem1/1(term), Product4/1  "term_ratio_out"
  Product4/1 -> Transfer Fcn/1
  Add3/1 -> F_friction/1
  Constant1/1 -> Bus Creator1/7  "sigma3"
  Constant2/1 -> Bus Creator/7  "sigma3"
  Constant3/1 -> Bus Creator1/8  "tau_L"
  Constant4/1 -> Bus Creator/8  "tau_L"
  [sigma3] -> Product8/1
  Product8/1 -> Add3/4
  [xc_dot_sim] -> Product9/2, Product9/3, Product9/1
  Product9/1 -> Product8/2
  Bus Selector/4 -> [sigma3]  "<sigma3>"
  xc_dot/1 -> [xc_dot_sim]
  Constant23/1 -> Bus Creator1/1  "Fc"
  Subsystem1/1(z) -> Scope2/1, Product4/2, [z], Unit Delay/1
  Switch1/1 -> [Params]
  Transfer Fcn/1 -> Add2/2

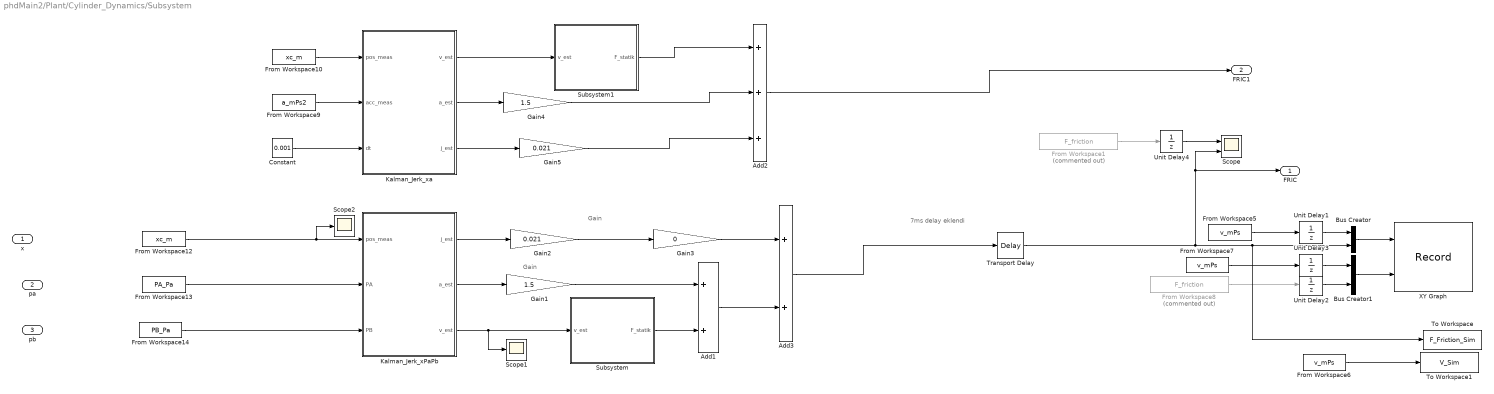
== system phdMain2/Plant/Cylinder_Dynamics/Subsystem ==
  note: Gain
  note: 7ms delay eklendi
  note: Gain
  x : Inport
  pa : Inport  Port=2
  pb : Inport  Port=3
  Add1 : Sum
  Add2 : Sum  Inputs=+++
  Add3 : Sum
  Bus Creator : BusCreator  Inputs=2
  Bus Creator1 : BusCreator  Inputs=2
  Constant : Constant  Value=0.001
  From Workspace1 : FromWorkspace  Commented=on  VariableName=F_friction
  From Workspace10 : FromWorkspace  VariableName=xc_m
  From Workspace12 : FromWorkspace  VariableName=xc_m
  From Workspace13 : FromWorkspace  VariableName=PA_Pa
  From Workspace14 : FromWorkspace  VariableName=PB_Pa
  From Workspace5 : FromWorkspace  VariableName=v_mPs
  From Workspace6 : FromWorkspace  VariableName=v_mPs
  From Workspace7 : FromWorkspace  VariableName=v_mPs
  From Workspace8 : FromWorkspace  Commented=on  VariableName=F_friction
  From Workspace9 : FromWorkspace  VariableName=a_mPs2
  Gain1 : Gain  Gain=1.5
  Gain2 : Gain  Gain=0.021
  Gain3 : Gain  Gain=0
  Gain4 : Gain  Gain=1.5
  Gain5 : Gain  Gain=0.021
  Kalman_Jerk_xPaPb : MATLAB Function  TreatAsAtomicUnit=on
  Kalman_Jerk_xa : MATLAB Function  TreatAsAtomicUnit=on
  Scope : Scope  NumInputPorts=2
  Scope1 : Scope
  Scope2 : Scope
  Subsystem : Subsystem
  Subsystem1 : Subsystem
  To Workspace : ToWorkspace  VariableName=F_Friction_Sim  SaveFormat=Timeseries  SampleTime=-1
  To Workspace1 : ToWorkspace  VariableName=V_Sim  SaveFormat=Timeseries  SampleTime=-1
  Transport Delay : TransportDelay  DelayTime=7e-3
  Unit Delay{1..4} (4 alike) : UnitDelay  SampleTime=-1  HasFrameUpgradeWarning=on
  XY Graph : Record  FileSettingsInternal="{\"entries\":[{\"content\":{\"excelSettings\":{\"content\":{},\"type\":\"Streamout.ExcelSettings\"}},\"type\":\"Streamout.FileSettingStorage\",\"uuid\":\"\"}],\"packageUris\":[\"http:\\/\\/schema.mathworks.com\\/mf0\\/streamout_blocks\\/R2020a\"],\"version\":\"1.0\"}"  Layout=[1 1]  SignalsInternal="{\"entries\":[{\"content\":{\"signals\":[{\"content\":{\"blockPath\":[],\"dimensions\":[1],\"domain\":\"\",\"lineColor\":\"#0072bd\",\"port\":1,\"signalID\":13135,\"signalName\":\"Bus Creator\"},\"type\":\"RecordBlkView.Signal\",\"uuid\":\"\"},{\"content\":{\"blockPath\":[],\"dimensions\":[1],\"domain\":\"\",\"lineColor\":\"#d95319\",\"port\":2,\"signalID\":13138,\"signalName\":\"Bus Creator1\"},\"type\":\"RecordBlkView.Signal\",\"uuid\":\"\"}]},\"type\":\"RecordBlkView.InputSignals\",\"uuid\":\"\"}],\"packageUris\":[\"http:\\/\\/schema.mathworks.com\\/mf0\\/streamout_blocks\\/R2020a\"],\"version\":\"1.0\"}"  VisualizationBindings="{\"xyplotplugin\":{\"info\":[{\"series\":[],\"subplotID\":1}]}}"  CompatibilityTag=XY
  FRIC : Outport
  FRIC1 : Outport  Port=2
  wires:
  Unit Delay2/1 -> Bus Creator1/2
  From Workspace9/1 -> Kalman_Jerk_xa/2(acc_meas)
  Constant/1 -> Kalman_Jerk_xa/3(dt)
  From Workspace12/1 -> Scope2/1, Kalman_Jerk_xPaPb/1(pos_meas)
  From Workspace7/1 -> Unit Delay3/1
  Unit Delay3/1 -> Bus Creator1/1
  From Workspace13/1 -> Kalman_Jerk_xPaPb/2(PA)
  Add3/1 -> Transport Delay/1
  Bus Creator1/1 -> XY Graph/2
  From Workspace10/1 -> Kalman_Jerk_xa/1(pos_meas)
  From Workspace5/1 -> Unit Delay1/1
  Bus Creator/1 -> XY Graph/1
  From Workspace14/1 -> Kalman_Jerk_xPaPb/3(PB)
  Kalman_Jerk_xPaPb/1(j_est) -> Gain2/1
  From Workspace8/1 -> Unit Delay2/1
  Kalman_Jerk_xPaPb/2(a_est) -> Gain1/1
  From Workspace6/1 -> To Workspace1/1
  Unit Delay1/1 -> Bus Creator/1
  Kalman_Jerk_xPaPb/3(v_est) -> Scope1/1, Subsystem/1(v_est)
  From Workspace1/1 -> Unit Delay4/1
  Unit Delay4/1 -> Scope/1
  Transport Delay/1 -> Scope/2, FRIC/1, Bus Creator/2, To Workspace/1
  Subsystem/1(F_statik) -> Add1/2
  Gain1/1 -> Add1/1
  Gain2/1 -> Gain3/1
  Add1/1 -> Add3/2
  Gain3/1 -> Add3/1
  Kalman_Jerk_xa/2(a_est) -> Gain4/1
  Kalman_Jerk_xa/1(v_est) -> Subsystem1/1(v_est)
  Subsystem1/1(F_statik) -> Add2/1
  Gain4/1 -> Add2/2
  Add2/1 -> FRIC1/1
  Kalman_Jerk_xa/3(j_est) -> Gain5/1
  Gain5/1 -> Add2/3

== system phdMain2/Plant/Cylinder_Dynamics/Subsystem1 ==
  Constant2 : Constant  Value=-0.09580
  Constant5 : Constant  Value=0.09580
  Constant6 : Constant  Value=1e6
  Constant7 : Constant  Value=2e-3
  MATLAB Function1 : MATLAB Function  TreatAsAtomicUnit=on
  F_end : Outport
  wires:
  Constant7/1 -> MATLAB Function1/6(v_lock)
  [xc_sim] -> MATLAB Function1/1(x)
  [xc_dot_sim] -> MATLAB Function1/2(x_dot)
  Constant6/1 -> MATLAB Function1/5(k_end)
  Constant2/1 -> MATLAB Function1/3(xmin)
  Constant5/1 -> MATLAB Function1/4(xmax)
  MATLAB Function1/1(F_end) -> F_end/1

== system phdMain2/Subsystem2/Subsystem3/Subsystem ==
  y : Inport
  phi2_hat : Inport  Port=2
  d1_hat : Inport  Port=3
  l1 : Inport  Port=4
  eta : Inport  Port=5
  phi1_hat : Inport  Port=6
  Add : Sum  Inputs=+-
  Add1 : Sum
  Add2 : Sum
  Product : Product
  Product1 : Product
  phi1_hat_dot : Outport
  wires:
  eta/1 -> Product/2
  l1/1 -> Product/1
  phi1_hat/1 -> Add/2
  y/1 -> Add/1
  Product/1 -> Product1/1
  Add/1 -> Product1/2
  Product1/1 -> Add1/2
  d1_hat/1 -> Add1/1
  Add1/1 -> Add2/2
  phi2_hat/1 -> Add2/1
  Add2/1 -> phi1_hat_dot/1

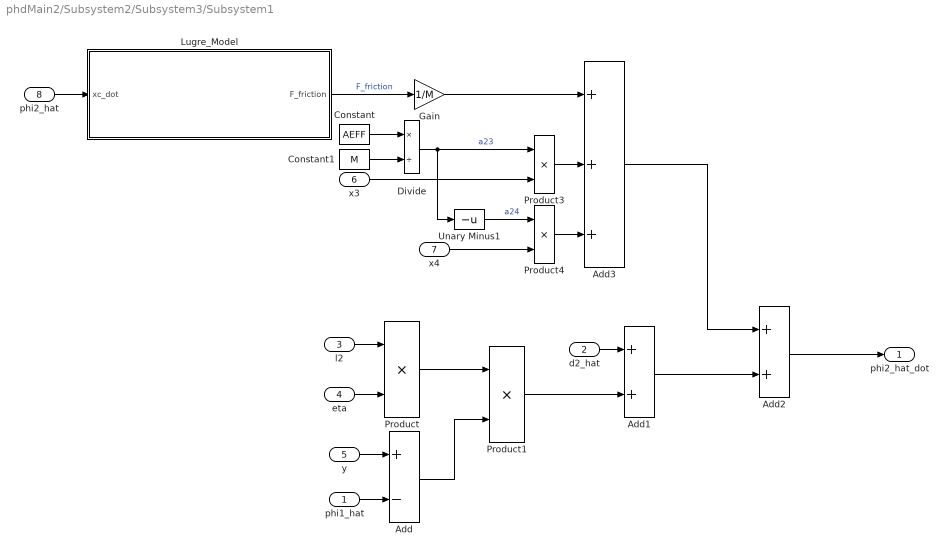
== system phdMain2/Subsystem2/Subsystem3/Subsystem1 ==
  phi1_hat : Inport
  d2_hat : Inport  Port=2
  l2 : Inport  Port=3
  eta : Inport  Port=4
  y : Inport  Port=5
  x3 : Inport  Port=6
  x4 : Inport  Port=7
  phi2_hat : Inport  Port=8
  Add : Sum  Inputs=+-
  Add1 : Sum
  Add2 : Sum
  Add3 : Sum  Inputs=+++
  Constant : Constant  Value=AEFF
  Constant1 : Constant  Value=M
  Divide : Product  Inputs=*/  RndMeth=Zero  SaturateOnIntegerOverflow=on
  Gain : Gain  Gain=1/M
  Lugre_Model : Subsystem
  Product{,1,3..4} (4 alike) : Product
  Unary Minus1 : UnaryMinus
  phi2_hat_dot : Outport
  wires:
  Add2/1 -> phi2_hat_dot/1
  Add1/1 -> Add2/2
  d2_hat/1 -> Add1/1
  Product1/1 -> Add1/2
  Add/1 -> Product1/2
  Product/1 -> Product1/1
  y/1 -> Add/1
  phi1_hat/1 -> Add/2
  l2/1 -> Product/1
  eta/1 -> Product/2
  Divide/1 -> Product3/1, Unary Minus1/1  "a23"
  x3/1 -> Product3/2
  Unary Minus1/1 -> Product4/1  "a24"
  x4/1 -> Product4/2
  Product3/1 -> Add3/2
  Product4/1 -> Add3/3
  Add3/1 -> Add2/1
  phi2_hat/1 -> Lugre_Model/1(xc_dot)
  Gain/1 -> Add3/1
  Lugre_Model/1(F_friction) -> Gain/1  "F_friction"
  Constant/1 -> Divide/1
  Constant1/1 -> Divide/2

== system phdMain2/Subsystem2/Subsystem3/Subsystem3 ==
  phi2_hat : Inport
  gamma1 : Inport  Port=2
  phi1_hat : Inport  Port=3
  sigma1_hat : Inport  Port=4
  Add : Sum
  Add1 : Sum
  Product : Product
  Product1 : Product
  Unary Minus : UnaryMinus
  sigma1_hat_dot : Outport
  wires:
  sigma1_hat/1 -> Add/1
  Product/1 -> Add/2
  Add/1 -> Add1/2
  phi2_hat/1 -> Add1/1
  gamma1/1 -> Unary Minus/1, Product/2
  phi1_hat/1 -> Product/1
  Add1/1 -> Product1/1
  Unary Minus/1 -> Product1/2
  Product1/1 -> sigma1_hat_dot/1

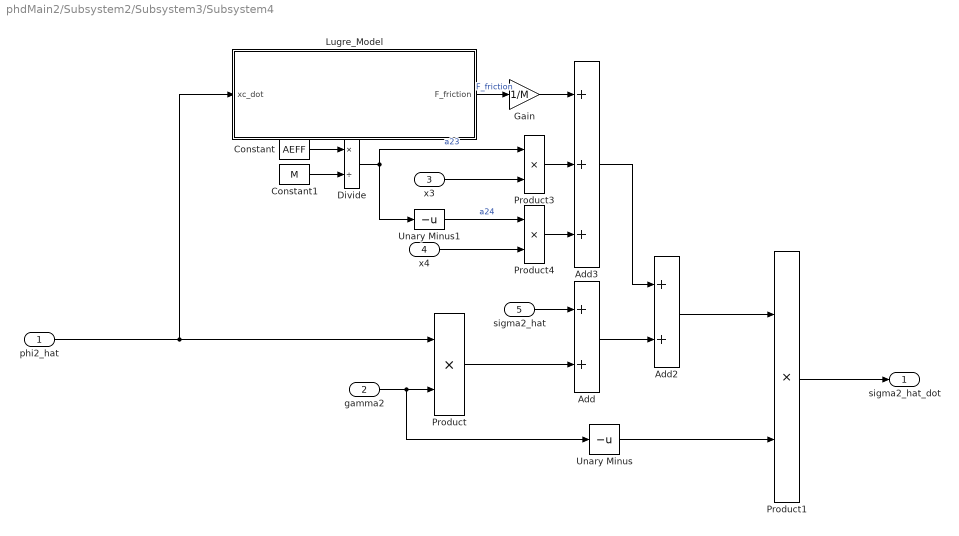
== system phdMain2/Subsystem2/Subsystem3/Subsystem4 ==
  phi2_hat : Inport
  gamma2 : Inport  Port=2
  x3 : Inport  Port=3
  x4 : Inport  Port=4
  sigma2_hat : Inport  Port=5
  Add : Sum
  Add2 : Sum
  Add3 : Sum  Inputs=+++
  Constant : Constant  Value=AEFF
  Constant1 : Constant  Value=M
  Divide : Product  Inputs=*/  RndMeth=Zero  SaturateOnIntegerOverflow=on
  Gain : Gain  Gain=1/M
  Lugre_Model : Subsystem
  Product{,1,3..4} (4 alike) : Product
  Unary Minus : UnaryMinus
  Unary Minus1 : UnaryMinus
  sigma2_hat_dot : Outport
  wires:
  Product1/1 -> sigma2_hat_dot/1
  gamma2/1 -> Unary Minus/1, Product/2
  Product/1 -> Add/2
  sigma2_hat/1 -> Add/1
  Product3/1 -> Add3/2
  Product4/1 -> Add3/3
  x4/1 -> Product4/2
  phi2_hat/1 -> Product/1, Lugre_Model/1(xc_dot)
  Unary Minus1/1 -> Product4/1  "a24"
  x3/1 -> Product3/2
  Add3/1 -> Add2/1
  Gain/1 -> Add3/1
  Add/1 -> Add2/2
  Add2/1 -> Product1/1
  Unary Minus/1 -> Product1/2
  Lugre_Model/1(F_friction) -> Gain/1  "F_friction"
  Constant/1 -> Divide/1
  Divide/1 -> Product3/1, Unary Minus1/1  "a23"
  Constant1/1 -> Divide/2

== system phdMain2/Subsystem2/Subsystem3/Subsystem6 ==
  sigma1_hat : Inport
  gamma1 : Inport  Port=2
  phi1_hat : Inport  Port=3
  Add : Sum
  Product : Product
  d1_hat : Outport
  wires:
  sigma1_hat/1 -> Add/1
  gamma1/1 -> Product/1
  phi1_hat/1 -> Product/2
  Product/1 -> Add/2
  Add/1 -> d1_hat/1

== system phdMain2/Subsystem2/Subsystem3/Subsystem7 ==
  sigma2_hat : Inport
  gamma2 : Inport  Port=2
  phi2_hat : Inport  Port=3
  Add : Sum
  Product : Product
  d2_hat : Outport
  wires:
  gamma2/1 -> Product/1
  sigma2_hat/1 -> Add/1
  Product/1 -> Add/2
  Add/1 -> d2_hat/1
  phi2_hat/1 -> Product/2

== system phdMain2/Plant/Cylinder_Dynamics/Lugre_Model/Subsystem1 ==
  term : Inport
  z_prev : Inport  Port=2
  v : Inport  Port=3
  Add : Sum
  Add1 : Sum
  Constant : Constant
  Gain : Gain  Gain=1e-3
  Gain1 : Gain  Gain=1e-3
  Math Reciprocal2 : Math  Operator=reciprocal  SignedPower=on
  Product : Product
  z : Outport
  wires:
  term/1 -> Gain1/1
  z_prev/1 -> Add/1
  v/1 -> Gain/1
  Gain/1 -> Add/2
  Add/1 -> Product/1
  Gain1/1 -> Add1/2
  Constant/1 -> Add1/1
  Add1/1 -> Math Reciprocal2/1
  Math Reciprocal2/1 -> Product/2
  Product/1 -> z/1

== system phdMain2/Plant/Cylinder_Dynamics/Subsystem/Subsystem ==
  v_est : Inport
  MATLAB Function : MATLAB Function  TreatAsAtomicUnit=on
  F_statik : Outport
  wires:
  v_est/1 -> MATLAB Function/1(v)
  MATLAB Function/1(F_statik) -> F_statik/1

== system phdMain2/Plant/Cylinder_Dynamics/Subsystem/Subsystem1 ==
  v_est : Inport
  MATLAB Function : MATLAB Function  TreatAsAtomicUnit=on
  F_statik : Outport
  wires:
  MATLAB Function/1(F_statik) -> F_statik/1
  v_est/1 -> MATLAB Function/1(v)

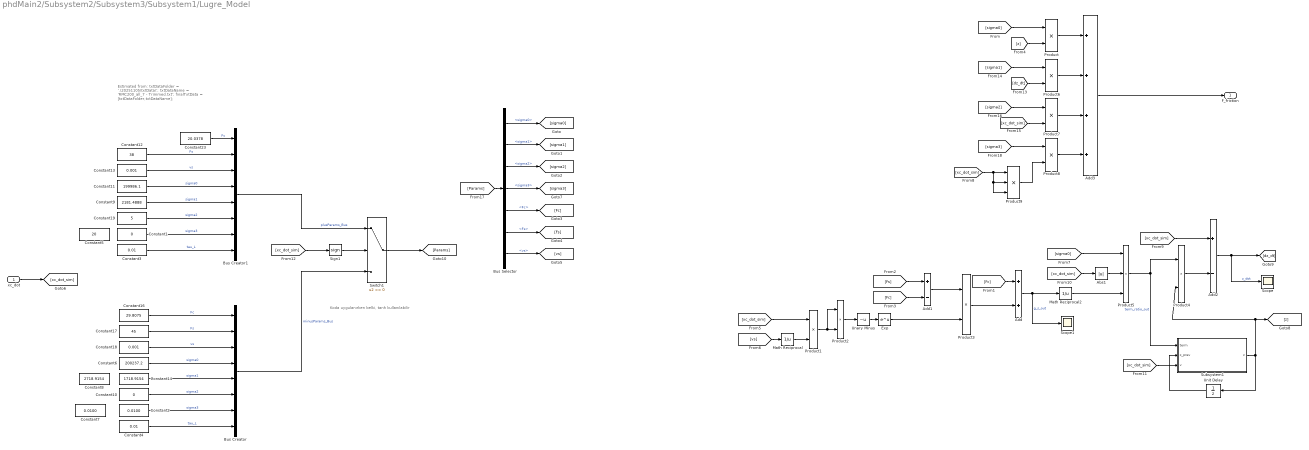
== system phdMain2/Subsystem2/Subsystem3/Subsystem1/Lugre_Model ==
  note: Koda uygulanırken belki, tanh kullanılabilir
  note: Estimated from:
      |
      | txtDataFolder = '.\20251105\txtData\';
      | txtDataName = 'RMC200_all_7 - Trimmed.txt';
      | finalTxtData = [txtDataFolder,txtDataName];
  xc_dot : Inport  OutDataTypeStr=double
  Abs1 : Abs  SaturateOnIntegerOverflow=off
  Add : Sum
  Add1 : Sum  Inputs=+-
  Add2 : Sum  Inputs=+-
  Add3 : Sum  Inputs=++++
  Bus Selector : BusSelector  OutputSignals=sigma0,sigma1,sigma2,sigma3,Fc,Fs,vs
  Bus Creator : BusCreator  Inputs=8
  Bus Creator1 : BusCreator  Inputs=8
  Constant1 : Constant  Value=0  OutDataTypeStr=double
  Constant10 : Constant  Value=0  OutDataTypeStr=double
  Constant11 : Constant  Value=199986.1  OutDataTypeStr=double
  Constant12 : Constant  Value=38  OutDataTypeStr=double
  Constant13 : Constant  Value=0.001  OutDataTypeStr=double
  Constant14 : Constant  Value=1718.9154  OutDataTypeStr=double
  Constant16 : Constant  Value=29.8075  OutDataTypeStr=double
  Constant17 : Constant  Value=45  OutDataTypeStr=double
  Constant18 : Constant  Value=0.001  OutDataTypeStr=double
  Constant19 : Constant  Value=5  OutDataTypeStr=double
  Constant2 : Constant  Value=0.0100  OutDataTypeStr=double
  Constant23 : Constant  Value=20.0378  OutDataTypeStr=double
  Constant3 : Constant  Value=0.01  OutDataTypeStr=double
  Constant4 : Constant  Value=0.01  OutDataTypeStr=double
  Constant5 : Constant  Value=20  OutDataTypeStr=double
  Constant6 : Constant  Value=200237.2  OutDataTypeStr=double
  Constant7 : Constant  Value=0.0100  OutDataTypeStr=double
  Constant8 : Constant  Value=2718.9154  OutDataTypeStr=double
  Constant9 : Constant  Value=2181.4888  OutDataTypeStr=double
  Exp : Math  SignedPower=on
  Math Reciprocal : Math  Operator=reciprocal  SignedPower=on
  Math Reciprocal2 : Math  Operator=reciprocal  SignedPower=on
  Product{,1..4,6..8} (8 alike) : Product
  Product5 : Product  Inputs=3
  Product9 : Product  Inputs=3
  Scope : Scope
  Scope1 : Scope
  Sign1 : Signum
  Subsystem1 : Subsystem
  Switch1 : Switch  SaturateOnIntegerOverflow=off  InputSameDT=off
  Unary Minus : UnaryMinus
  Unit Delay : UnitDelay  SampleTime=-1  HasFrameUpgradeWarning=on
  F_friction : Outport
  wires:
  Constant18/1 -> Bus Creator/3  "vs"
  Constant13/1 -> Bus Creator1/3  "vs"
  Constant12/1 -> Bus Creator1/2  "Fs"
  Constant17/1 -> Bus Creator/2  "Fs"
  Constant14/1 -> Bus Creator/5  "sigma1"
  Constant6/1 -> Bus Creator/4  "sigma0"
  Constant10/1 -> Bus Creator/6  "sigma2"
  Constant16/1 -> Bus Creator/1  "Fc"
  Constant9/1 -> Bus Creator1/5  "sigma1"
  Constant11/1 -> Bus Creator1/4  "sigma0"
  Constant19/1 -> Bus Creator1/6  "sigma2"
  Product7/1 -> Add3/3
  Product6/1 -> Add3/2
  [sigma2] -> Product7/1
  [xc_dot_sim] -> Product7/2
  [dz_dt] -> Product6/2
  [sigma1] -> Product6/1
  Product/1 -> Add3/1
  [z] -> Product/2
  [sigma0] -> Product5/1
  Abs1/1 -> Product5/2
  Add/1 -> Math Reciprocal2/1, Scope1/1  "g_s_out"
  [xc_dot_sim] -> Abs1/1
  Add1/1 -> Product3/1
  Unary Minus/1 -> Exp/1
  Product2/1 -> Unary Minus/1
  Product1/1 -> Product2/2, Product2/1
  [xc_dot_sim] -> Product1/1
  Math Reciprocal/1 -> Product1/2
  [vs] -> Math Reciprocal/1
  [Fc] -> Add1/2
  [Fs] -> Add1/1
  [Fc] -> Add/1
  [sigma0] -> Product/1
  Product3/1 -> Add/2
  [xc_dot_sim] -> Sign1/1
  Bus Creator1/1 -> Switch1/1  "plusParams_Bus"
  Bus Creator/1 -> Switch1/3  "minusParams_Bus"
  Switch1/1 -> [Params]
  [Params] -> Bus Selector/1
  Bus Selector/1 -> [sigma0]  "<sigma0>"
  Bus Selector/2 -> [sigma1]  "<sigma1>"
  Bus Selector/3 -> [sigma2]  "<sigma2>"
  Bus Selector/5 -> [Fc]  "<Fc>"
  Bus Selector/6 -> [Fs]  "<Fs>"
  Bus Selector/7 -> [vs]  "<vs>"
  Math Reciprocal2/1 -> Product5/3
  Exp/1 -> Product3/2
  Add2/1 -> Scope/1, [dz_dt]  "z_dot"
  Sign1/1 -> Switch1/2
  [xc_dot_sim] -> Add2/1
  Subsystem1/1(z) -> Product4/2, [z], Unit Delay/1
  [xc_dot_sim] -> Subsystem1/3(v)
  Unit Delay/1 -> Subsystem1/2(z_prev)
  Product5/1 -> Subsystem1/1(term), Product4/1  "term_ratio_out"
  Product4/1 -> Add2/2
  Add3/1 -> F_friction/1
  Constant1/1 -> Bus Creator1/7  "sigma3"
  Constant2/1 -> Bus Creator/7  "sigma3"
  Constant3/1 -> Bus Creator1/8  "tau_L"
  Constant4/1 -> Bus Creator/8  "tau_L"
  [sigma3] -> Product8/1
  Product8/1 -> Add3/4
  [xc_dot_sim] -> Product9/2, Product9/3, Product9/1
  Product9/1 -> Product8/2
  Bus Selector/4 -> [sigma3]  "<sigma3>"
  xc_dot/1 -> [xc_dot_sim]
  Constant23/1 -> Bus Creator1/1  "Fc"

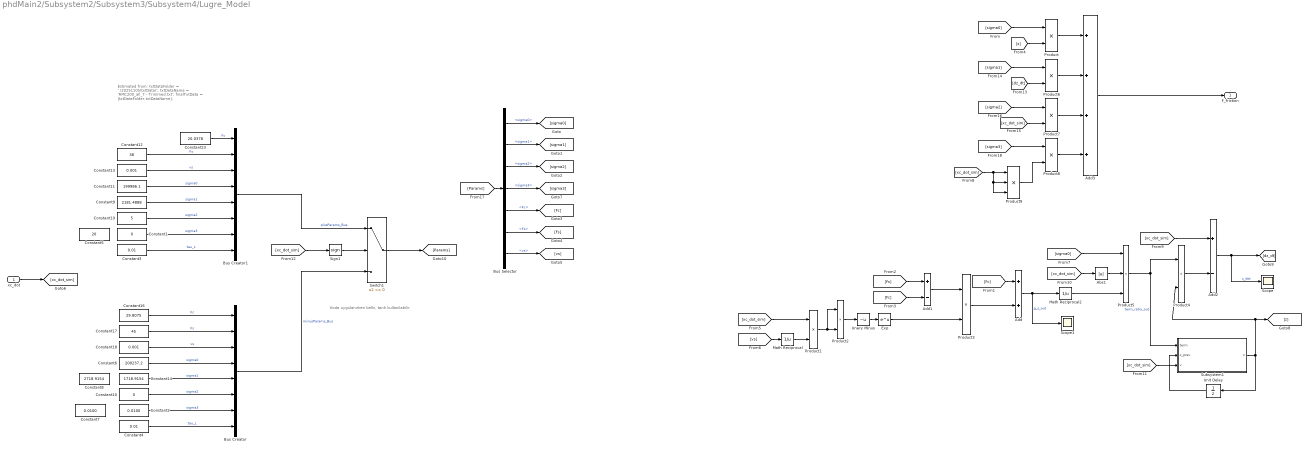
== system phdMain2/Subsystem2/Subsystem3/Subsystem4/Lugre_Model ==
  note: Koda uygulanırken belki, tanh kullanılabilir
  note: Estimated from:
      |
      | txtDataFolder = '.\20251105\txtData\';
      | txtDataName = 'RMC200_all_7 - Trimmed.txt';
      | finalTxtData = [txtDataFolder,txtDataName];
  xc_dot : Inport  OutDataTypeStr=double
  Abs1 : Abs  SaturateOnIntegerOverflow=off
  Add : Sum
  Add1 : Sum  Inputs=+-
  Add2 : Sum  Inputs=+-
  Add3 : Sum  Inputs=++++
  Bus Selector : BusSelector  OutputSignals=sigma0,sigma1,sigma2,sigma3,Fc,Fs,vs
  Bus Creator : BusCreator  Inputs=8
  Bus Creator1 : BusCreator  Inputs=8
  Constant1 : Constant  Value=0  OutDataTypeStr=double
  Constant10 : Constant  Value=0  OutDataTypeStr=double
  Constant11 : Constant  Value=199986.1  OutDataTypeStr=double
  Constant12 : Constant  Value=38  OutDataTypeStr=double
  Constant13 : Constant  Value=0.001  OutDataTypeStr=double
  Constant14 : Constant  Value=1718.9154  OutDataTypeStr=double
  Constant16 : Constant  Value=29.8075  OutDataTypeStr=double
  Constant17 : Constant  Value=45  OutDataTypeStr=double
  Constant18 : Constant  Value=0.001  OutDataTypeStr=double
  Constant19 : Constant  Value=5  OutDataTypeStr=double
  Constant2 : Constant  Value=0.0100  OutDataTypeStr=double
  Constant23 : Constant  Value=20.0378  OutDataTypeStr=double
  Constant3 : Constant  Value=0.01  OutDataTypeStr=double
  Constant4 : Constant  Value=0.01  OutDataTypeStr=double
  Constant5 : Constant  Value=20  OutDataTypeStr=double
  Constant6 : Constant  Value=200237.2  OutDataTypeStr=double
  Constant7 : Constant  Value=0.0100  OutDataTypeStr=double
  Constant8 : Constant  Value=2718.9154  OutDataTypeStr=double
  Constant9 : Constant  Value=2181.4888  OutDataTypeStr=double
  Exp : Math  SignedPower=on
  Math Reciprocal : Math  Operator=reciprocal  SignedPower=on
  Math Reciprocal2 : Math  Operator=reciprocal  SignedPower=on
  Product{,1..4,6..8} (8 alike) : Product
  Product5 : Product  Inputs=3
  Product9 : Product  Inputs=3
  Scope : Scope
  Scope1 : Scope
  Sign1 : Signum
  Subsystem1 : Subsystem
  Switch1 : Switch  SaturateOnIntegerOverflow=off  InputSameDT=off
  Unary Minus : UnaryMinus
  Unit Delay : UnitDelay  SampleTime=-1  HasFrameUpgradeWarning=on
  F_friction : Outport
  wires:
  Constant18/1 -> Bus Creator/3  "vs"
  Constant13/1 -> Bus Creator1/3  "vs"
  Constant12/1 -> Bus Creator1/2  "Fs"
  Constant17/1 -> Bus Creator/2  "Fs"
  Constant14/1 -> Bus Creator/5  "sigma1"
  Constant6/1 -> Bus Creator/4  "sigma0"
  Constant10/1 -> Bus Creator/6  "sigma2"
  Constant16/1 -> Bus Creator/1  "Fc"
  Constant9/1 -> Bus Creator1/5  "sigma1"
  Constant11/1 -> Bus Creator1/4  "sigma0"
  Constant19/1 -> Bus Creator1/6  "sigma2"
  Product7/1 -> Add3/3
  Product6/1 -> Add3/2
  [sigma2] -> Product7/1
  [xc_dot_sim] -> Product7/2
  [dz_dt] -> Product6/2
  [sigma1] -> Product6/1
  Product/1 -> Add3/1
  [z] -> Product/2
  [sigma0] -> Product5/1
  Abs1/1 -> Product5/2
  Add/1 -> Math Reciprocal2/1, Scope1/1  "g_s_out"
  [xc_dot_sim] -> Abs1/1
  Add1/1 -> Product3/1
  Unary Minus/1 -> Exp/1
  Product2/1 -> Unary Minus/1
  Product1/1 -> Product2/2, Product2/1
  [xc_dot_sim] -> Product1/1
  Math Reciprocal/1 -> Product1/2
  [vs] -> Math Reciprocal/1
  [Fc] -> Add1/2
  [Fs] -> Add1/1
  [Fc] -> Add/1
  [sigma0] -> Product/1
  Product3/1 -> Add/2
  [xc_dot_sim] -> Sign1/1
  Bus Creator1/1 -> Switch1/1  "plusParams_Bus"
  Bus Creator/1 -> Switch1/3  "minusParams_Bus"
  Switch1/1 -> [Params]
  [Params] -> Bus Selector/1
  Bus Selector/1 -> [sigma0]  "<sigma0>"
  Bus Selector/2 -> [sigma1]  "<sigma1>"
  Bus Selector/3 -> [sigma2]  "<sigma2>"
  Bus Selector/5 -> [Fc]  "<Fc>"
  Bus Selector/6 -> [Fs]  "<Fs>"
  Bus Selector/7 -> [vs]  "<vs>"
  Math Reciprocal2/1 -> Product5/3
  Exp/1 -> Product3/2
  Add2/1 -> Scope/1, [dz_dt]  "z_dot"
  Sign1/1 -> Switch1/2
  [xc_dot_sim] -> Add2/1
  Subsystem1/1(z) -> Product4/2, [z], Unit Delay/1
  [xc_dot_sim] -> Subsystem1/3(v)
  Unit Delay/1 -> Subsystem1/2(z_prev)
  Product5/1 -> Subsystem1/1(term), Product4/1  "term_ratio_out"
  Product4/1 -> Add2/2
  Add3/1 -> F_friction/1
  Constant1/1 -> Bus Creator1/7  "sigma3"
  Constant2/1 -> Bus Creator/7  "sigma3"
  Constant3/1 -> Bus Creator1/8  "tau_L"
  Constant4/1 -> Bus Creator/8  "tau_L"
  [sigma3] -> Product8/1
  Product8/1 -> Add3/4
  [xc_dot_sim] -> Product9/2, Product9/3, Product9/1
  Product9/1 -> Product8/2
  Bus Selector/4 -> [sigma3]  "<sigma3>"
  xc_dot/1 -> [xc_dot_sim]
  Constant23/1 -> Bus Creator1/1  "Fc"
